simulink model "r2sdf_fft_bb"  (R2019a)
settings: Solver=VariableStepAuto  StartTime=0.0  StopTime=10.0  RelTol=1e-3
libraries: xbsIndex_r4 x2, xps_library x1
settings Model: Creator=talon  LastModifiedBy=talon

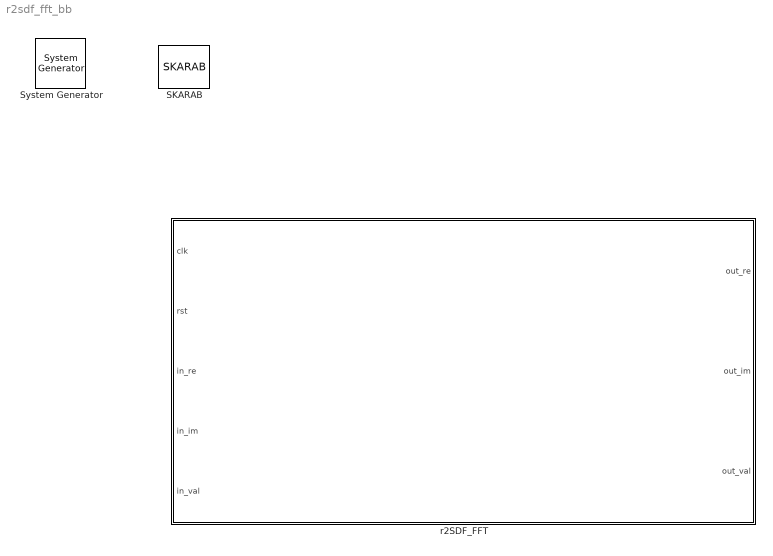
== system r2sdf_fft_bb ==
  " System Generator" : xbsIndex_r4/ System Generator  Tag=genX  xilinxfamily=kintex7  part=xc7k325t  speed=-3  package=fbg676  synthesis_tool=Vivado  clock_wrapper=Clock Enables  directory=./netlist  proj_type=Vivado  Synth_file=Vivado Synthesis Defaults  Impl_file=Vivado Implementation Defaults  testbench=off  simulink_period=1  sysclk_period=10  dcm_input_clock_period=10  incr_netlist=off  trim_vbits=Everywhere in SubSystem  dbl_ovrd=According to Block Masks  core_generation=According to Block Masks  run_coregen=off  deprecated_control=off  eval_field=0  block_type=sysgen
  SKARAB : xps_library/Platforms/SKARAB  Tag=xps:xsg  hw_sys=SKARAB:xc7vx690t  clk_src=sys_clk  clk_rate=156.25  sample_period=1  synthesis_tool=XST
      settings: SourceProductName=CASPER XPS Blockset
  r2SDF_FFT : Subsystem  mask{g_nof_chan=1024, g_use_reorder=on, g_in_dat_w=8, g_out_dat_w=14, g_stage_dat_w=14, g_guard_w=2, g_nof_points=0}
      mask prompts: g_nof_chan "Number of channels"; g_use_reorder "Reorder output"; g_in_dat_w "Input data width"; g_out_dat_w "Output data width"; g_stage_dat_w "Stage data width"; g_guard_w "Guard bit width"; g_nof_points "Number of points"

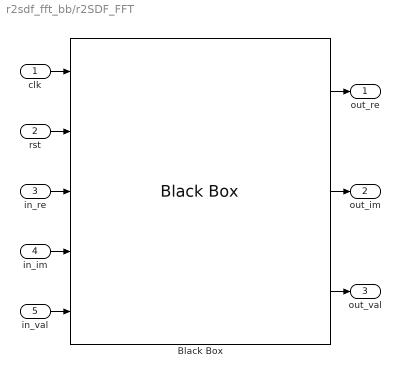
== system r2sdf_fft_bb/r2SDF_FFT ==
  clk : Inport
  rst : Inport  Port=2
  in_re : Inport  Port=3
  in_im : Inport  Port=4
  in_val : Inport  Port=5
  Black Box : xbsIndex_r4/Black Box  init_code=rTwoSDF_config  sim_method=ISE Simulator  verbose=off  block_type=blackbox2
  out_re : Outport
  out_im : Outport  Port=2
  out_val : Outport  Port=3
  wires:
  in_val/1 -> Black Box/5
  rst/1 -> Black Box/2
  Black Box/2 -> out_im/1
  in_im/1 -> Black Box/4
  in_re/1 -> Black Box/3
  Black Box/1 -> out_re/1
  clk/1 -> Black Box/1
  Black Box/3 -> out_val/1
